simulink model "RemoteVehicleModel_Callas"  (R2018b)
settings: Solver=ode1  StartTime=0.0  StopTime=inf  FixedStep=0.0005  MaxStep=0.001  RelTol=1e-3
libraries: simulink x2, dspnetwork x1
settings Model: Creator=mhewat  LastModifiedBy=llacroix
settings SolverCC: AutoInsertRateTranBlk=on
settings DataIOCC: LimitDataPoints=on  SaveFormat=Array  SignalLoggingSaveFormat=ModelDataLogs
settings OptimizationCC: ExpressionDepthLimit=2147483647  InitFltsAndDblsToZero=on  LifeSpan=1
settings DebuggingCC: UnderspecifiedInitializationDetection=Classic  MergeDetectMultiDrivingBlocksExec=none  SolverPrmCheckMsg=warning  MultiTaskRateTransMsg=warning  ParameterDowncastMsg=warning  FcnCallInpInsideContextMsg=warning  StateNameClashWarn=warning  SFUnexpectedBacktrackingDiag=warning  SFNoUnconditionalDefaultTransitionDiag=warning  SFExecutionAtInitializationDiag=none
settings HardwareCC: ProdBitPerPointer=32  ProdBitPerSizeT=32  ProdBitPerPtrDiffT=32  ProdLargestAtomicFloat=None  ProdIntDivRoundTo=Undefined  ProdEndianess=Unspecified  ProdWordSize=32  ProdHWDeviceType=32-bit Generic
settings ModelReferenceCC: PropagateSignalLabelsOutOfModel=off
settings SFSimCC: SimUseLocalCustomCode=off  SimParseCustomCode=off  MATLABDynamicMemAlloc=off
settings RTWCC: SystemTargetFile=ert.tlc  TemplateMakefile=ert_default_tmf  Description=Real-Time Workshop Embedded Coder (no auto configuration)  RTWUseLocalCustomCode=off  CustomInclude=../../../include  TargetLang=C++
settings RTWCC: CustomSource=|
  | source/ComVhcDynHelper.cpp
  | source/cal_reseau_win32.cpp
  | source/cal_timer_win32.cpp
settings CodeAppCC: IgnoreCustomStorageClasses=off  CustomSymbolStrType=$N$R$M  StateflowObjectComments=on  InternalIdentifier=Classic
settings ERTTargetCC: MultiwordLength=2048  GenerateSampleERTMain=on  SupportComplex=off  SupportContinuousTime=on  SupportNonInlinedSFcns=on  ERTCustomFileTemplate=example_file_process.tlc  ConvertIfToSwitch=off  SuppressUnreachableDefaultCases=off
settings ConfigComp: CovMetricSettings=dw  CovHtmlReporting=on  CovSaveCumulativeToWorkspaceVar=on  CovSaveSingleToWorkspaceVar=on  CovExternalEMLEnable=off

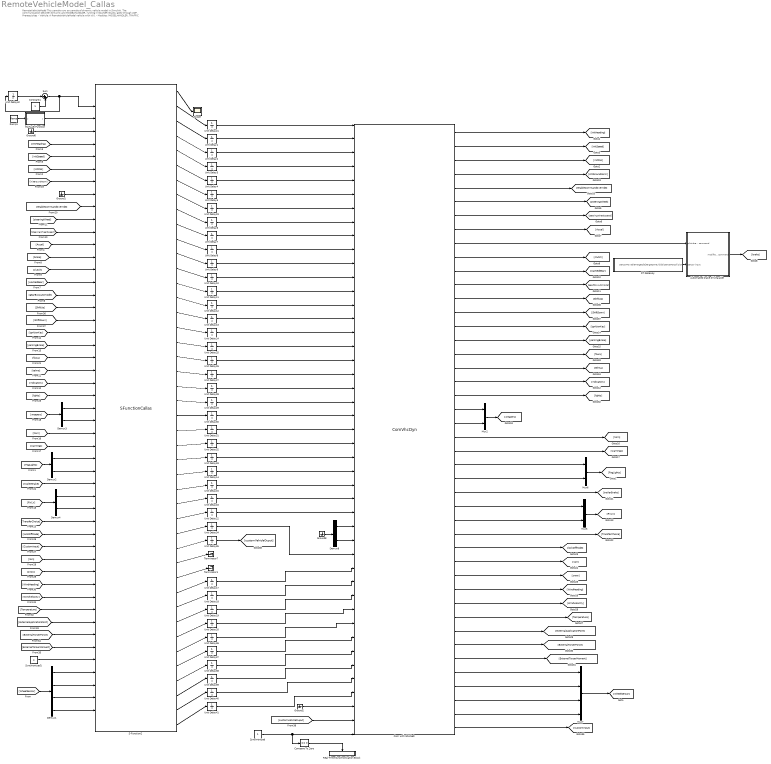
== system RemoteVehicleModel_Callas ==
  note: RemoteVehicleModel
      | This sample runs an sample of dynamic vehicle model in Simulink. The communication between Simulink and MODELHANDLER, running in SCANeR Studio, goes through UDP.
      |
      | Prerequisites
      | - Vehicle: A RemoteVehicleModel vehicle with id 0.
      | - Modules: MODELHANDLER, TRAFFIC
  Automated brake driving aide : Subsystem
  Com with SCANeR : S-Function  InitFcn=try, set_param(gcb,'FunctionName','ComVhcDyn'), end  FunctionName=ComVhcDyn  SFunctionModules=ComVhcDyn_wrapper ComVhcDynHelper cal_reseau_win32 cal_timer_win32  SFunctionDeploymentMode=off  EnableBusSupport=off  mask(S-Function Builder){}
      mask help: The S-Function Builder block creates a wrapper C-MEX S-function from your supplied C code with multiple input ports, output ports, and a variable number of scalar, vector, or matrix parameters. The input and output ports can propagate Simulink built-in data types, fixed-point datatypes, complex, frame, 1-D, and 2-D signals. This block also supports discrete and continuous states of type real. You can optionally have the block generate a TLC file to be used with Real-Time Workshop for code generation.
      mask init:
      | val = [[.9  0.75 0.75 1 1 .9 .9 1]',[1 1 0.75 0.75 .9 .9 1 .9]'];try , sys = get_param(gcb,'SfunBuilderFcnName');if isempty(sys), sys = get_param(gcb,'FunctionName'); end,catch, sys = get_param(gcb,'FunctionName'); end
      settings: CopyFcn=set_param(gcbh,'LinkStatus','none')  PreSaveFcn=try, set_param(gcb,'FunctionName','ComVhcDyn'), end  OpenFcn=sfunctionwizard(gcbh)
      mask Display: plot(val(:,1),val(:,2)),disp(sys), port_label('input',1,'pos'), port_label('input',2,'roll'), port_label('input',3,'pitch'), port_label('input',4,'heading'), port_label('input',5,'speed'), port_label('input',6,'accel'), port_label('input',7,'engineStatus'), port_label('input',8,'engineSpeed'), port_label('input',9,'effectiveSteeringWheelAngle'), port_label('input',10,'SteeringWheelFeedbackTorque'), port_label('input',11,'effectiveGasPedalPos'), port_label('input',12,'effectiveBrake'), port_label('input',13,'effectiveHandBrake'), port_label('input',14,'effectiveClutch'), port_label('input',15,'effectiveGearEngaged'), port_label('input',16,'effectiveGearBoxMode'), port_label('input',17,'effectiveIgnitionKeyPosition'), port_label('input',18,'effectiveConsumption'), port_label('input',19,'isEngineRetarder'), port_label('input',20,'effectiveBrakeRetarderNotch'), port_label('input',21,'effectiveTrailerBrake'), port_label('input',22,'effectiveTransferChoice'), port_label('input',23,'effectiveLockDiffMode'), port_label('input',24,'effectiveForceLockup'), port_label('input',25,'effectivePlowMode'), port_label('input',26,'effectiveHorn'), port_label('input',27,'effectiveLights'), port_label('input',28,'effectiveRearWiperState'), port_label('input',29,'effectiveFrontWiperState'), port_label('input',30,'reserved1'), port_label('input',31,'reserved2'), port_label('input',32,'effectiveBatteryStateOfCharge'), port_label('input',33,'wheel0'), port_label('input',34,'wheel1'), port_label('input',35,'wheel2'), port_label('input',36,'wheel3'), port_label('input',37,'electricMotor0'), port_label('input',38,'electricMotor1'), port_label('input',39,'electricMotor2'), port_label('input',40,'electricMotor3'), port_label('input',41,'electricMotor4'), port_label('input',42,'electricMotor5'), port_label('input',43,'electricMotor6'), port_label('input',44,'customVehicleOutput'), port_label('input',45,'synchronizedValue'), port_label('output',1,'initHeading'), port_label('output',2,'initSpeed'), port_label('output',3,'initGroundPos'), port_label('output',4,'initGroundNorm'), port_label('output',5,'enableCommandOverride'), port_label('output',6,'steeringWheel'), port_label('output',7,'steeringWheelSpeed'), port_label('output',8,'accelerator'), port_label('output',9,'brake'), port_label('output',10,'clutch'), port_label('output',11,'wantedGear'), port_label('output',12,'gearBoxAutoMode'), port_label('output',13,'shiftUp'), port_label('output',14,'shiftDown'), port_label('output',15,'ignitionKey'), port_label('output',16,'parkingBrake'), port_label('output',17,'fowa'), port_label('output',18,'telma'), port_label('output',19,'indicators'), port_label('output',20,'lights'), port_label('output',21,'rearWiperState'), port_label('output',22,'frontWiperState'), port_label('output',23,'horn'), port_label('output',24,'warnings'), port_label('output',25,'frontFogLights'), port_label('output',26,'rearFogLights'), port_label('output',27,'trailerBrake'), port_label('output',28,'rVLVState'), port_label('output',29,'rVLVTarget'), port_label('output',30,'transferChoice'), port_label('output',31,'lockDiffMode'), port_label('output',32,'rain'), port_label('output',33,'snow'), port_label('output',34,'windHeading'), port_label('output',35,'windVelocity'), port_label('output',36,'temperature'), port_label('output',37,'externalTorserApplicationPoint'), port_label('output',38,'externalTorserForce'), port_label('output',39,'externalTorserMoment'), port_label('output',40,'wheelSensor0'), port_label('output',41,'wheelSensor1'), port_label('output',42,'wheelSensor2'), port_label('output',43,'wheelSensor3'), port_label('output',44,'customVehicleInput')
  Compare To Zero : simulink/Logic and Bit Operations/Compare To Zero  relop===  OutDataTypeStr=boolean  ZeroCross=off
  Constant1 : Constant
  Demux1 : Demux
  Demux{2..4,8} (4 alike) : Demux  Outputs=2
  Ground{1..2,6,8} (4 alike) : Ground
  MATLAB Function : MATLAB Function  TreatAsAtomicUnit=on
  Mux2 : Mux  Inputs=2
  Mux5 : Mux  Inputs=2
  Mux6 : Mux  Inputs=2
  Mux7 : Mux
  RT Gateway : Subsystem
  Ramp1 : simulink/Sources/Ramp  slope=1  start=1  InitialOutput=0
  Real-Time Synchronization Block : Subsystem  TreatAsAtomicUnit=on
  S-Function2 : S-Function  FunctionName=SFunctionCallas  SFunctionDeploymentMode=off  EnableBusSupport=off
      mask Display:
      | disp(['SFunctionCallas'])
      | port_label('input', 1, 'packetNumber')
      | port_label('input', 2, 'simulationMode')
      | port_label('input', 3, 'options')
      | port_label('input', 4, 'initHeading')
      | port_label('input', 5, 'initSpeed')
      | port_label('input', 6, 'initGroundPos')
      | port_label('input', 7, 'initGroundNorm')
      | 
      | port_label('input', 8, 'scANeRTime')
      | port_label('input', 9, 'isCommandOverride')
      | 
      | port_label('input', 10, 'steeringWheel')
      | port_label('input', 11, 'steeringWheelSpeed')
      | port_label('input', 12, 'accelerator')
      | port_label('input', 13, 'brake')
      | port_label('input', 14, 'clutch')
      | port_label('input', 15, 'wantedGear')
      | port_label('input', 16, 'gearBoxAutoMode')
      | port_label('input', 17, 'shiftUp')
      | port_label('input', 18, 'shiftDown')
      | port_label('input', 19, 'ignitionKey')
      | port_label('input', 20, 'parkingBrake')
      | port_label('input', 21, 'fowa')
      | port_label('input', 22, 'telma')
      | port_label('input', 23, 'indicator')
      | port_label('input', 24, 'lights')
      | port_label('input', 25, 'rearWiperState')
      | port_label('input', 26, 'frontWiperState')
      | port_label('input', 27, 'horn')
      | port_label('input', 28, 'warnings')
      | port_label('input', 29, 'frontFogLights')
      | port_label('input', 30, 'rearFogLights')
      | port_label('input', 31, 'trailerBrake')
      | port_label('input', 32, 'rVLVState')
      | port_label('input', 33, 'rVLVTarget')
      | port_label('input', 34, 'transferChoice')
      | port_label('input', 35, 'lockDiffMode')
      | port_label('input', 36, 'customVehicleInputs')
      | port_label('input', 37, 'rain')
      | port_label('input', 38, 'snow')
      | port_label('input', 39, 'windHeading')
      | port_label('input', 40, 'windVelocity')
      | port_label('input', 41, 'temperature')
      | port_label('input', 42, 'externalTorserApplicationPoint')
      | port_label('input', 43, 'externalTorserForce')
      | port_label('input', 44, 'externalTorserMoment')
      | port_label('input', 45, 'numberOfContactPoints')
      | port_label('input', 46, 'wheelState1')
      | port_label('input', 47, 'wheelState2')
      | port_label('input', 48, 'wheelState3')
      | port_label('input', 49, 'wheelState4')
      | 
      | port_label('output', 1, 'packetNumber')
      | port_label('output', 2, 'pos')
      | port_label('output', 3, 'roll')
      | port_label('output', 4, 'pitch')
      | port_label('output', 5, 'heading')
      | port_label('output', 6, 'speed')
      | port_label('output', 7, 'accel')
      | port_label('output', 8, 'engineStatus')
      | port_label('output', 9, 'engineSpeed')
      | 
      | port_label('output', 10, 'effectiveSteeringWheelAngle')
      | port_label('output', 11, 'SteeringWheelFeedbackTorque')
      | port_label('output', 12, 'effectiveGasPedalPos')
      | 
      | port_label('output', 13, 'effectiveBrake')
      | port_label('output', 14, 'effectiveHandBrake')
      | port_label('output', 15, 'effectiveClutch')
      | port_label('output', 16, 'effectiveGearEngaged')
      | port_label('output', 17, 'effectiveGearBoxMode')
      | 
      | port_label('output', 18, 'effectiveIgnitionKeyPosition')
      | port_label('output', 19, 'effectiveConsumption')
      | port_label('output', 20, 'isEngineRetarder')
      | port_label('output', 21, 'effectiveBrakeRetarderNotch')
      | port_label('output', 22, 'effectiveTrailerBrake')
      | port_label('output', 23, 'effectiveTransferChoice')
      | port_label('output', 24, 'effectiveLockDiffMode')
      | port_label('output', 25, 'effectiveForceLockup')
      | port_label('output', 26, 'effectivePlowMode')
      | port_label('output', 27, 'effectiveHorn')
      | port_label('output', 28, 'effectiveLights')
      | port_label('output', 29,'effectiveRearWiperState')
      | port_label('output', 30, 'effectiveFrontWiperState')
      | port_label('output', 31, 'effectiveBatteryStateOfCharge')
      | port_label('output', 32, 'customVehicleOutput')
      | port_label('output', 33, 'electricMotorNumber')
      | port_label('output', 34, 'wheelNumber')
      | 
      | port_label('output', 35, 'wheelState1')
      | port_label('output', 36, 'wheelState2')
      | port_label('output', 37, 'wheelState3')
      | port_label('output', 38, 'wheelState4')
      | port_label('output', 39, 'electricMotor1')
      | port_label('output', 40, 'electricMotor2')
      | port_label('output', 41, 'electricMotor3')
      | port_label('output', 42, 'electricMotor4')
      | port_label('output', 43, 'electricMotor5')
      | port_label('output', 44, 'electricMotor6')
  Scope : Scope
  Sum : Sum  Inputs=|++
  Synchronized : Constant
  Synchronized1 : Constant  Value=4
  Terminator1 : Terminator
  Terminator7 : Terminator
  Unit Delay{1..42} (42 alike) : UnitDelay  SampleTime=-1
  wires:
  Unit Delay1/1 -> Com with SCANeR/2
  Unit Delay2/1 -> Com with SCANeR/3
  Unit Delay3/1 -> Com with SCANeR/4
  Unit Delay4/1 -> Com with SCANeR/5
  Unit Delay5/1 -> Com with SCANeR/6
  Unit Delay6/1 -> Com with SCANeR/8
  Unit Delay7/1 -> Com with SCANeR/9
  Unit Delay8/1 -> Com with SCANeR/10
  Unit Delay9/1 -> Com with SCANeR/11
  Unit Delay10/1 -> Com with SCANeR/12
  Unit Delay11/1 -> Com with SCANeR/13
  Unit Delay12/1 -> Com with SCANeR/14
  Unit Delay13/1 -> Com with SCANeR/15
  Unit Delay21/1 -> Com with SCANeR/1
  Synchronized/1 -> Com with SCANeR/45, Compare To Zero/1
  Compare To Zero/1 -> Real-Time Synchronization Block/Enable
  Com with SCANeR/21 -> Mux2/1
  Com with SCANeR/22 -> Mux2/2
  RT Gateway/1(SensorMovableTargets[0]/targetsArray[0]/distanceToCollision) -> Automated brake driving aide/2(sensor input)
  Com with SCANeR/9 -> Automated brake driving aide/1(pilot brake command)
  [WheelSensor] -> Demux1/1
  [FogLights] -> Demux2/1
  [initSpeed] -> S-Function2/5
  [RVLV] -> Demux4/1
  [initHeading] -> S-Function2/4
  [initPos] -> S-Function2/6
  Com with SCANeR/18 -> [telma]
  Com with SCANeR/1 -> [initHeading]
  Com with SCANeR/2 -> [initSpeed]
  Com with SCANeR/3 -> [initPos]
  Com with SCANeR/6 -> [steeringWheel]
  Com with SCANeR/7 -> [steeringWheelSpeed]
  Com with SCANeR/8 -> [Accel]
  Automated brake driving aide/1("modified brake command ") -> [brake]
  Com with SCANeR/10 -> [clutch]
  Com with SCANeR/11 -> [wantedGear]
  Com with SCANeR/12 -> [gearBoxAutomode]
  Com with SCANeR/15 -> [ignitionKey]
  Com with SCANeR/16 -> [parkingBrake]
  Com with SCANeR/17 -> [fowa]
  Com with SCANeR/19 -> [indicators]
  Com with SCANeR/28 -> Mux5/1
  Com with SCANeR/29 -> Mux5/2
  Mux7/1 -> [WheelSensor]
  Mux6/1 -> [FogLights]
  Mux5/1 -> [RVLV]
  Com with SCANeR/26 -> Mux6/2
  Com with SCANeR/23 -> [horn]
  Com with SCANeR/25 -> Mux6/1
  Com with SCANeR/24 -> [warnings]
  Mux2/1 -> [weapers]
  Demux8/1 -> Com with SCANeR/30
  Demux8/2 -> Com with SCANeR/31
  Ground8/1 -> Demux8/1
  Com with SCANeR/20 -> [lights]
  Com with SCANeR/4 -> [initGroundNorm]
  Com with SCANeR/27 -> [trailerBrake]
  Com with SCANeR/40 -> Mux7/1
  Com with SCANeR/41 -> Mux7/2
  Com with SCANeR/42 -> Mux7/3
  Com with SCANeR/43 -> Mux7/4
  [initGroundNorm] -> S-Function2/7
  Com with SCANeR/5 -> [EnableCommandOverride]
  [steeringWheelSpeed] -> S-Function2/11
  [Accel] -> S-Function2/12
  [wantedGear] -> S-Function2/15
  [gearBoxAutomode] -> S-Function2/16
  [brake] -> S-Function2/13
  [clutch] -> S-Function2/14
  [parkingBrake] -> S-Function2/20
  [ignitionKey] -> S-Function2/19
  Com with SCANeR/30 -> [TransferChoice]
  Com with SCANeR/31 -> [lockDiffMode]
  Com with SCANeR/32 -> [rain]
  Com with SCANeR/33 -> [snow]
  Com with SCANeR/34 -> [WindHeading]
  Com with SCANeR/35 -> [WindVelocity]
  Com with SCANeR/37 -> [ExternalApplicationPoint]
  Com with SCANeR/36 -> [Temperature]
  Com with SCANeR/38 -> [ExternalTorserForce]
  Com with SCANeR/39 -> [ExternalTorserMoment]
  Com with SCANeR/44 -> [CustomInput]
  Ground6/1 -> S-Function2/3
  [weapers] -> Demux3/1
  Com with SCANeR/13 -> [ShiftUp]
  Com with SCANeR/14 -> [ShiftDown]
  [ShiftUp] -> S-Function2/17
  [ShiftDown] -> S-Function2/18
  S-Function2/2 -> Unit Delay21/1
  S-Function2/3 -> Unit Delay1/1
  S-Function2/4 -> Unit Delay2/1
  S-Function2/5 -> Unit Delay3/1
  S-Function2/6 -> Unit Delay4/1
  S-Function2/7 -> Unit Delay5/1
  S-Function2/8 -> Unit Delay23/1
  S-Function2/9 -> Unit Delay6/1
  S-Function2/10 -> Unit Delay7/1
  S-Function2/11 -> Unit Delay8/1
  S-Function2/12 -> Unit Delay9/1
  S-Function2/13 -> Unit Delay10/1
  S-Function2/14 -> Unit Delay11/1
  S-Function2/15 -> Unit Delay12/1
  S-Function2/16 -> Unit Delay13/1
  Unit Delay23/1 -> Com with SCANeR/7
  S-Function2/17 -> Unit Delay24/1
  S-Function2/18 -> Unit Delay25/1
  S-Function2/19 -> Unit Delay26/1
  S-Function2/20 -> Unit Delay27/1
  S-Function2/21 -> Unit Delay28/1
  S-Function2/22 -> Unit Delay29/1
  S-Function2/23 -> Unit Delay30/1
  S-Function2/24 -> Unit Delay31/1
  S-Function2/25 -> Unit Delay32/1
  S-Function2/26 -> Unit Delay33/1
  S-Function2/27 -> Unit Delay14/1
  S-Function2/28 -> Unit Delay15/1
  S-Function2/29 -> Unit Delay16/1
  S-Function2/30 -> Unit Delay22/1
  S-Function2/31 -> Unit Delay34/1
  S-Function2/35 -> Unit Delay17/1
  S-Function2/36 -> Unit Delay18/1
  S-Function2/37 -> Unit Delay19/1
  S-Function2/38 -> Unit Delay20/1
  S-Function2/39 -> Unit Delay36/1
  S-Function2/40 -> Unit Delay37/1
  S-Function2/41 -> Unit Delay38/1
  S-Function2/42 -> Unit Delay39/1
  S-Function2/43 -> Unit Delay40/1
  S-Function2/44 -> Unit Delay41/1
  S-Function2/33 -> Terminator7/1
  S-Function2/34 -> Terminator1/1
  S-Function2/32 -> Unit Delay35/1
  Ground2/1 -> Com with SCANeR/43
  Unit Delay24/1 -> Com with SCANeR/16
  Unit Delay25/1 -> Com with SCANeR/17
  Unit Delay26/1 -> Com with SCANeR/18
  Unit Delay34/1 -> Com with SCANeR/32
  Unit Delay35/1 -> [customVehicleOuput]
  S-Function2/1 -> Scope/1
  Ramp1/1 -> MATLAB Function/1(u)
  MATLAB Function/1(y) -> S-Function2/2
  Unit Delay17/1 -> Com with SCANeR/33
  Unit Delay18/1 -> Com with SCANeR/34
  Unit Delay19/1 -> Com with SCANeR/35
  Synchronized1/1 -> S-Function2/45
  Unit Delay20/1 -> Com with SCANeR/36
  Demux1/1 -> S-Function2/46
  Demux1/2 -> S-Function2/47
  Demux1/3 -> S-Function2/48
  Demux1/4 -> S-Function2/49
  [steeringWheel] -> S-Function2/10
  [fowa] -> S-Function2/21
  [telma] -> S-Function2/22
  [indicators] -> S-Function2/23
  [lights] -> S-Function2/24
  Demux3/1 -> S-Function2/25
  Demux3/2 -> S-Function2/26
  [horn] -> S-Function2/27
  [warnings] -> S-Function2/28
  Demux2/1 -> S-Function2/29
  Demux2/2 -> S-Function2/30
  [trailerBrake] -> S-Function2/31
  Demux4/1 -> S-Function2/32
  Demux4/2 -> S-Function2/33
  [TransferChoice] -> S-Function2/34
  [lockDiffMode] -> S-Function2/35
  [CustomInput] -> S-Function2/36
  [rain] -> S-Function2/37
  [snow] -> S-Function2/38
  [WindHeading] -> S-Function2/39
  [WindVelocity] -> S-Function2/40
  [Temperature] -> S-Function2/41
  [ExternalApplicationPoint] -> S-Function2/42
  [ExternalTorserForce] -> S-Function2/43
  [ExternalTorserMoment] -> S-Function2/44
  Unit Delay27/1 -> Com with SCANeR/19
  Unit Delay28/1 -> Com with SCANeR/20
  Unit Delay29/1 -> Com with SCANeR/21
  Unit Delay30/1 -> Com with SCANeR/22
  Unit Delay31/1 -> Com with SCANeR/23
  Unit Delay32/1 -> Com with SCANeR/24
  Unit Delay33/1 -> Com with SCANeR/25
  Unit Delay14/1 -> Com with SCANeR/26
  Unit Delay15/1 -> Com with SCANeR/27
  Unit Delay16/1 -> Com with SCANeR/28
  Unit Delay22/1 -> Com with SCANeR/29
  Unit Delay36/1 -> Com with SCANeR/37
  Unit Delay37/1 -> Com with SCANeR/38
  Unit Delay38/1 -> Com with SCANeR/39
  Unit Delay39/1 -> Com with SCANeR/40
  Unit Delay40/1 -> Com with SCANeR/41
  Unit Delay41/1 -> Com with SCANeR/42
  [customVehicleOuput] -> Com with SCANeR/44
  [EnableCommandOverride] -> S-Function2/9
  Ground1/1 -> S-Function2/8
  Constant1/1 -> Sum/2
  Sum/1 -> Unit Delay42/1, S-Function2/1
  Unit Delay42/1 -> Sum/1

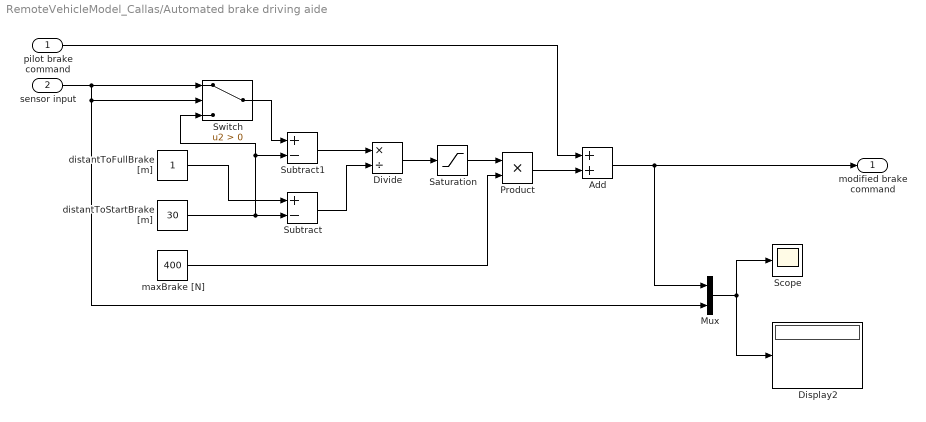
== system RemoteVehicleModel_Callas/Automated brake driving aide ==
  pilot brake command : Inport
  sensor input : Inport  Port=2
  Add : Sum
  Display2 : Display
  Divide : Product  Inputs=*/
  Mux : Mux  Inputs=2
  Product : Product
  Saturation : Saturate  UpperLimit=1  LowerLimit=0
  Scope : Scope
  Subtract : Sum  Inputs=+-
  Subtract1 : Sum  Inputs=+-
  Switch : Switch  Criteria=u2 > Threshold
  distantToFullBrake [m] : Constant
  distantToStartBrake [m] : Constant  Value=30
  maxBrake [N] : Constant  Value=400
  "modified brake command " : Outport
  wires:
  Add/1 -> "modified brake command "/1, Mux/1
  sensor input/1 -> Switch/2, Mux/2, Switch/1
  pilot brake command/1 -> Add/1
  distantToFullBrake [m]/1 -> Subtract/1
  distantToStartBrake [m]/1 -> Switch/3, Subtract1/2, Subtract/2
  Mux/1 -> Scope/1, Display2/1
  Subtract/1 -> Divide/2
  maxBrake [N]/1 -> Product/2
  Subtract1/1 -> Divide/1
  Divide/1 -> Saturation/1
  Saturation/1 -> Product/1
  Product/1 -> Add/2
  Switch/1 -> Subtract1/1

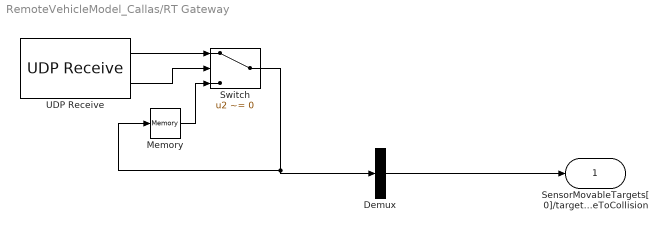
== system RemoteVehicleModel_Callas/RT Gateway ==
  Demux : Demux  Outputs=1
  Memory : Memory  InheritSampleTime=on
  Switch : Switch  Criteria=u2 ~= 0
  UDP Receive : dspnetwork/UDP Receive  localURL='0.0.0.0'  localPort=8192  remoteURL='0.0.0.0'  remotePort=-1  recvBufferSize=8  dims=1  signalDatatype=double  isVarSize=off  showBlockingTime=on  blockingTime=0  sampletime=0.002  blockPlatform=HOST
      settings: SourceProductName=DSP System Toolbox  SourceProductBaseCode=DS
  SensorMovableTargets[0]/targetsArray[0]/distanceToCollision : Outport
  wires:
  UDP Receive/1 -> Switch/1
  Demux/1 -> SensorMovableTargets[0]/targetsArray[0]/distanceToCollision/1
  UDP Receive/2 -> Switch/2
  Switch/1 -> Memory/1, Demux/1
  Memory/1 -> Switch/3

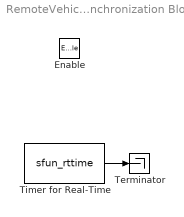
== system RemoteVehicleModel_Callas/Real-Time Synchronization Block ==
  Enable : EnablePort
  Terminator : Terminator
  Timer for Real-Time : S-Function  FunctionName=sfun_rttime  Parameters=1  SFunctionDeploymentMode=off  EnableBusSupport=off
  wires:
  Timer for Real-Time/1 -> Terminator/1

== matlab function RemoteVehicleModel_Callas/MATLAB Function ==
  data: u input; y output
function y = fcn(u)
if(u<5)
    y = 1;
else
    y= 2;
end
